simulink library "bcm"  (R2021b)
settings: Solver=VariableStepAuto  StartTime=0.0  StopTime=10.0  RelTol=1e-3
undefined symbols (not defined in the file or in its folder): ENUM_ANTITHEFT_ALARM, ENUM_ANTITHEFT_ARM, ENUM_ANTITHEFT_DISARM, ENUM_ANTITHEFT_WAIT, ENUM_GEARPOSNTOCAN_P, ENUM_PDKEYRAWLULOCK_INUNLOCK, ENUM_PDKEYRAWPS_INPS, ENUM_POWERSTA_READY, ENUM_POWERSTA_STANDBY, FALSE, KBCM_ALMBrightnessDark_enum, KBCM_AmbBlue_enum, KBCM_AmbBreathT_K, KBCM_AmbBreathTOut_K, KBCM_AmbGreen_enum, KBCM_AmbLightUser_enum, KBCM_AmbPreset_enum, KBCM_AmbRed_enum, KBCM_Antitheft_enum_ovrdflg, KBCM_Antitheft_enum_ovrdval, KBCM_APMDoorCtrlSta_flg_ovrdflg, KBCM_APMDoorCtrlSta_flg_ovrdval, KBCM_DelayTSW_flg, KBCM_DiagFLTC_mA, KBCM_DiagFMHT_s, KBCM_DiagFRTC_mA, KBCM_DiagRLTC_mA, KBCM_DiagRRTC_mA, KBCM_DrAPMRetryTimes_cnt, KBCM_DrOpenWdwOT_s, KBCM_DrOpenWdwReady_s, KBCM_ESSOffT_ms, KBCM_ESSOnT_ms, KBCM_IVIRstHoldT_ms, KBCM_IVIRstTriggerT_ms, KBCM_ONDelayT_ms, KBCM_ReDetectT_K, KBCM_RmLampKeep_min, KBCM_RmLpKeyInT_s, KBCM_RmLpKeyMissT_s, KBCM_SlpDebounceTime_s, KBCM_SPTGDetectT_sec, KBCM_SPTGLeave_flg, KBCM_SPTGLeftBound_cm, KBCM_SPTGLeftBoundOut_cm, KBCM_SPTGLowerBound_cm, KBCM_SPTGLowerBoundOut_cm, KBCM_SPTGRightBound_cm, KBCM_SPTGRightBoundOut_cm, KBCM_SPTGTOut_K, KBCM_SPTGUpperBound_cm, KBCM_SPTGUpperBoundOut_cm, KBCM_SPTGWaitDKC_sec, KBCM_USSDis_cm, KBCM_USSFilterT_K, KBCM_WaitAPMPwr_K, KBCM_WdwManualDetT_s, MIN2SEC, TRUE, XX2KXX
libraries: simulink x41, $bdroot x3, hcu_lib x2
(part 4 of 6)

== system bcm/BCM/BCM/FlasherSignal/Subsystem ==
  VINP_APSActive_flg : Inport
  VINP_AVMparkingmode_enum : Inport  Port=2
  Compare To Constant1 : simulink/Logic and Bit Operations/Compare To Constant  relop===  const=1  OutDataTypeStr=boolean
  Compare To Constant10 : simulink/Logic and Bit Operations/Compare To Constant  relop=>=  const=2  OutDataTypeStr=boolean
  Compare To Constant11 : simulink/Logic and Bit Operations/Compare To Constant  relop===  const=1  OutDataTypeStr=boolean
  Compare To Constant2 : simulink/Logic and Bit Operations/Compare To Constant  relop===  const=3  OutDataTypeStr=boolean
  Compare To Constant3 : simulink/Logic and Bit Operations/Compare To Constant  relop===  const=5  OutDataTypeStr=boolean
  Compare To Constant4 : simulink/Logic and Bit Operations/Compare To Constant  relop===  const=2  OutDataTypeStr=boolean
  Compare To Constant5 : simulink/Logic and Bit Operations/Compare To Constant  relop===  const=4  OutDataTypeStr=boolean
  Compare To Constant6 : simulink/Logic and Bit Operations/Compare To Constant  relop===  const=6  OutDataTypeStr=boolean
  Constant : Constant  OutDataTypeStr=uint8
  Constant1 : Constant  Value=0  OutDataTypeStr=uint8
  Constant2 : Constant  Value=2  OutDataTypeStr=uint8
  Constant3 : Constant  Value=0  OutDataTypeStr=uint8
  Constant7 : Constant  Value=0  OutDataTypeStr=uint8
  Detect Decrease : simulink/Logic and Bit Operations/Detect Decrease  vinit=0.0  OutDataTypeStr=boolean
  Detect Increase : simulink/Logic and Bit Operations/Detect Increase  vinit=0.0  OutDataTypeStr=boolean
  OR : Logic  Operator=OR  Inputs=3  AllPortsSameDT=off  OutDataTypeStr=boolean
  OR1 : Logic  Operator=OR  Inputs=3  AllPortsSameDT=off  OutDataTypeStr=boolean
  Sum : Sum  Inputs=|++
  Switch{,1..2,5} (4 alike) : Switch  Criteria=u2 > Threshold
  Unit Delay1 : UnitDelay  SampleTime=-1  HasFrameUpgradeWarning=on
  APS_LTurnReq : Outport
  APS_RTurnReq : Outport  Port=2
  wires:
  Compare To Constant2/1 -> OR/2
  Compare To Constant1/1 -> OR/1
  Compare To Constant3/1 -> OR/3
  Compare To Constant4/1 -> OR1/1
  Compare To Constant5/1 -> OR1/2
  Compare To Constant6/1 -> OR1/3
  Detect Increase/1 -> Switch/2
  OR/1 -> Switch1/2
  OR1/1 -> Switch2/2
  Constant/1 -> Switch1/1
  Constant1/1 -> Switch1/3
  Constant2/1 -> Switch2/1
  Constant3/1 -> Switch2/3
  Switch1/1 -> Sum/1
  Switch2/1 -> Sum/2
  Detect Decrease/1 -> Switch5/2
  Constant7/1 -> Switch5/1
  Switch5/1 -> Switch/3
  Unit Delay1/1 -> Switch5/3
  Switch/1 -> Compare To Constant10/1, Compare To Constant11/1, Unit Delay1/1
  Sum/1 -> Switch/1
  Compare To Constant10/1 -> APS_LTurnReq/1
  Compare To Constant11/1 -> APS_RTurnReq/1
  VINP_AVMparkingmode_enum/1 -> Compare To Constant6/1, Compare To Constant5/1, Compare To Constant4/1, Compare To Constant3/1, Compare To Constant2/1, Compare To Constant1/1
  VINP_APSActive_flg/1 -> Detect Decrease/1, Detect Increase/1

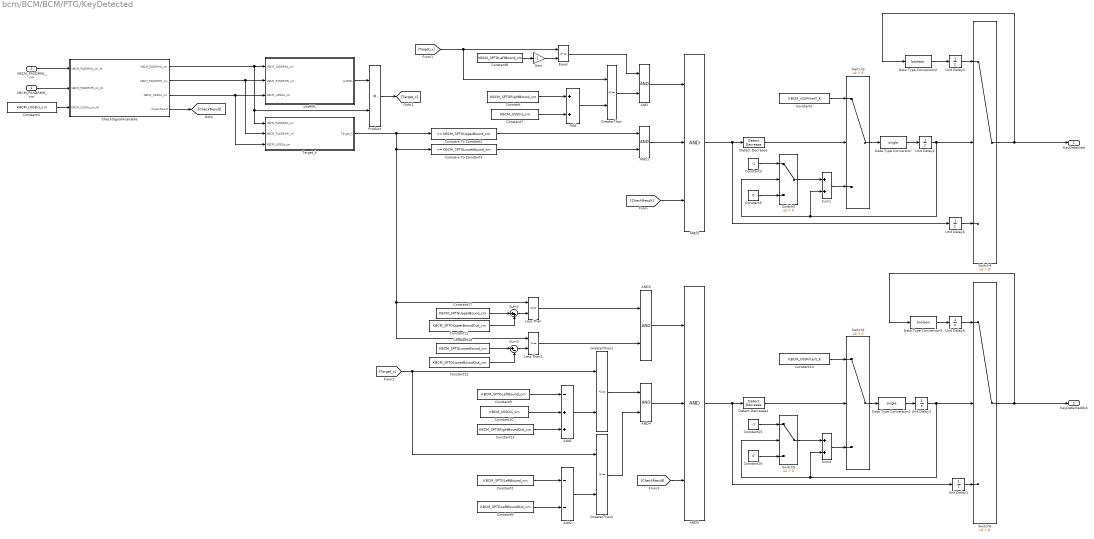
== system bcm/BCM/BCM/PTG/KeyDetected ==
  VBCM_PASDRMR_cm : Inport
  VBCM_PASDRML_cm : Inport  Port=2
  AND{,1,3..4} (4 alike) : Logic  AllPortsSameDT=off  OutDataTypeStr=boolean
  AND2 : Logic  Inputs=3  AllPortsSameDT=off  OutDataTypeStr=boolean
  AND5 : Logic  Inputs=3  AllPortsSameDT=off  OutDataTypeStr=boolean
  Add : Sum
  Add1 : Sum  Inputs=-++
  Add2 : Sum  Inputs=--
  CheckSignalAvailable : Subsystem
  Compare To Constant2 : simulink/Logic and Bit Operations/Compare To Constant  relop=<=  const=KBCM_SPTGUpperBound_cm  OutDataTypeStr=boolean
  Compare To Constant3 : simulink/Logic and Bit Operations/Compare To Constant  relop=>=  const=KBCM_SPTGLowerBound_cm  OutDataTypeStr=boolean
  Constant : Constant  Value=KBCM_SPTGRightBound_cm
  Constant1 : Constant  Value=KBCM_USSFilterT_K
  Constant10 : Constant  Value=KBCM_USSDis_cm
  Constant11 : Constant  Value=KBCM_SPTGUpperBoundOut_cm
  Constant12 : Constant  Value=KBCM_SPTGLowerBoundOut_cm
  Constant13 : Constant  Value=KBCM_SPTGRightBoundOut_cm
  Constant14 : Constant  Value=KBCM_USSFilterT_K
  Constant15 : Constant  Value=-1  OutDataTypeStr=single
  Constant16 : Constant  Value=0  OutDataTypeStr=single
  Constant17 : Constant  Value=KBCM_SPTGUpperBound_cm
  Constant18 : Constant  Value=KBCM_SPTGLowerBound_cm
  Constant2 : Constant  Value=KBCM_SPTGLeftBound_cm
  Constant3 : Constant  Value=-1  OutDataTypeStr=single
  Constant4 : Constant  Value=KBCM_USSDis_cm
  Constant5 : Constant  Value=0  OutDataTypeStr=single
  Constant6 : Constant  Value=KBCM_SPTGLeftBoundOut_cm
  Constant7 : Constant  Value=KBCM_USSDis_cm
  Constant8 : Constant  Value=KBCM_SPTGLeftBound_cm
  Constant9 : Constant  Value=KBCM_SPTGLeftBound_cm
  Data Type Conversion : DataTypeConversion  OutDataTypeStr=single
  Data Type Conversion1 : DataTypeConversion  OutDataTypeStr=single
  Data Type Conversion2 : DataTypeConversion  OutDataTypeStr=boolean
  Data Type Conversion3 : DataTypeConversion  OutDataTypeStr=boolean
  Detect Decrease : simulink/Logic and Bit Operations/Detect Decrease  vinit=0.0  OutDataTypeStr=boolean
  Detect Decrease1 : simulink/Logic and Bit Operations/Detect Decrease  vinit=0.0  OutDataTypeStr=boolean
  Equal : RelationalOperator  OutDataTypeStr=boolean  RndMeth=Simplest
  Gain : Gain  Gain=-1
  GreaterThan : RelationalOperator  Operator=<=  OutDataTypeStr=boolean  RndMeth=Simplest
  GreaterThan1 : RelationalOperator  Operator=<=  OutDataTypeStr=boolean  RndMeth=Simplest
  GreaterThan2 : RelationalOperator  OutDataTypeStr=boolean  RndMeth=Simplest
  Less Than : RelationalOperator  Operator=<=  OutDataTypeStr=boolean  RndMeth=Simplest
  Less Than1 : RelationalOperator  OutDataTypeStr=boolean  RndMeth=Simplest
  Product : Product
  Sum1 : Sum
  Sum2 : Sum  Inputs=|++
  Sum3 : Sum  Inputs=|+-
  Sum4 : Sum
  Switch{1..6} (6 alike) : Switch  Criteria=u2 > Threshold
  Target_h : Subsystem
  Unit Delay{1..6} (6 alike) : UnitDelay  SampleTime=-1  HasFrameUpgradeWarning=on
  cosRML : Subsystem
  KeyDetected : Outport
  KeyDetectedOut : Outport  Port=2
  wires:
  Constant4/1 -> CheckSignalAvailable/3(KBCM_USSDis_cm_IN)
  CheckSignalAvailable/1(VBCM_PASDRML_cm) -> cosRML/1(VBCM_PASDRML_cm), Target_h/1(VBCM_PASDRML_cm), Product/2
  CheckSignalAvailable/2(VBCM_PASDRMR_cm) -> Target_h/2(VBCM_PASDRMR_cm), cosRML/2(VBCM_PASDRMR_cm)
  CheckSignalAvailable/3(KBCM_USSDis_cm) -> Target_h/3(KBCM_USSDis_cm), cosRML/3(KBCM_USSDis_cm)
  Target_h/1(Target_h) -> Less Than1/1, Less Than/1, Compare To Constant3/1, Compare To Constant2/1
  Compare To Constant2/1 -> AND1/1
  Compare To Constant3/1 -> AND1/2
  AND1/1 -> AND2/2
  AND/1 -> AND2/1
  cosRML/1(cosRML) -> Product/1
  CheckSignalAvailable/4(CheckResult) -> [CheckResult]
  [CheckResult] -> AND2/3
  Detect Decrease/1 -> Switch2/2
  Switch2/1 -> Data Type Conversion/1
  Constant1/1 -> Switch2/1
  Sum1/1 -> Switch2/3
  Unit Delay2/1 -> Switch3/2, Sum1/2, Switch4/2
  Constant3/1 -> Switch3/1
  Constant5/1 -> Switch3/3
  Switch3/1 -> Sum1/1
  Switch4/1 -> Data Type Conversion2/1, KeyDetected/1
  Unit Delay4/1 -> Switch4/1
  VBCM_PASDRML_cm/1 -> CheckSignalAvailable/1(VBCM_PASDRML_cm_IN)
  VBCM_PASDRMR_cm/1 -> CheckSignalAvailable/2(VBCM_PASDRMR_cm_IN)
  AND2/1 -> Unit Delay6/1, Detect Decrease/1
  GreaterThan1/1 -> AND4/1
  Add1/1 -> GreaterThan1/2
  [Target_x] -> GreaterThan2/1, GreaterThan1/1
  Product/1 -> [Target_x]
  [Target_x] -> GreaterThan/1, Equal/1
  Constant17/1 -> Sum2/1
  Constant11/1 -> Sum2/2
  Constant12/1 -> Sum3/2
  Constant18/1 -> Sum3/1
  [CheckResult] -> AND5/3
  AND3/1 -> AND5/1
  AND4/1 -> AND5/2
  AND5/1 -> Unit Delay1/1, Detect Decrease1/1
  Unit Delay5/1 -> Switch6/1
  Switch6/1 -> KeyDetectedOut/1, Data Type Conversion3/1
  Switch5/1 -> Sum4/1
  Constant16/1 -> Switch5/3
  Constant15/1 -> Switch5/1
  Unit Delay3/1 -> Switch6/2, Sum4/2, Switch5/2
  Sum4/1 -> Switch1/3
  Constant14/1 -> Switch1/1
  Switch1/1 -> Data Type Conversion1/1
  Detect Decrease1/1 -> Switch1/2
  Sum2/1 -> Less Than/2
  Less Than/1 -> AND3/1
  Sum3/1 -> Less Than1/2
  Less Than1/1 -> AND3/2
  Constant10/1 -> Add1/2
  Constant9/1 -> Add1/1
  Constant13/1 -> Add1/3
  Constant7/1 -> Add/2
  Equal/1 -> AND/1
  GreaterThan/1 -> AND/2
  Constant/1 -> Add/1
  Add/1 -> GreaterThan/2
  GreaterThan2/1 -> AND4/2
  Constant2/1 -> Add2/1
  Constant6/1 -> Add2/2
  Add2/1 -> GreaterThan2/2
  Unit Delay1/1 -> Switch6/3
  Unit Delay6/1 -> Switch4/3
  Constant8/1 -> Gain/1
  Gain/1 -> Equal/2
  Data Type Conversion/1 -> Unit Delay2/1
  Data Type Conversion1/1 -> Unit Delay3/1
  Data Type Conversion2/1 -> Unit Delay4/1
  Data Type Conversion3/1 -> Unit Delay5/1

== system bcm/BCM/BCM/PTG/Subsystem1 ==
  VAPM_PASDRMR_cm : Inport
  Add4 : Sum
  Compare To Constant1 : simulink/Logic and Bit Operations/Compare To Constant  relop=~=  const=0  OutDataTypeStr=boolean
  Compare To Constant6 : simulink/Logic and Bit Operations/Compare To Constant  relop===  const=0  OutDataTypeStr=boolean
  Compare To Constant8 : simulink/Logic and Bit Operations/Compare To Constant  relop===  const=255  OutDataTypeStr=boolean
  Constant1 : Constant  Value=0  OutDataTypeStr=uint8
  Constant12 : Constant  OutDataTypeStr=uint8
  Constant13 : Constant  Value=0  OutDataTypeStr=uint8
  Constant2 : Constant  OutDataTypeStr=uint8
  Constant3 : Constant  Value=KBCM_SPTGTOut_K
  Constant4 : Constant  Value=255  OutDataTypeStr=uint8
  Constant5 : Constant  Value=KBCM_SPTGTOut_K
  Detect Change : simulink/Logic and Bit Operations/Detect Change  vinit=0  OutDataTypeStr=boolean
  Equal : RelationalOperator  OutDataTypeStr=boolean  RndMeth=Simplest
  Equal1 : RelationalOperator  Operator===  OutDataTypeStr=boolean  RndMeth=Simplest
  Equal2 : RelationalOperator  Operator=~=  OutDataTypeStr=boolean  RndMeth=Simplest
  Logical Operator : Logic  Inputs=3  AllPortsSameDT=off  OutDataTypeStr=boolean
  Logical Operator2 : Logic  Operator=OR  AllPortsSameDT=off  OutDataTypeStr=boolean
  Switch{2..3,8..9} (4 alike) : Switch  Criteria=u2 > Threshold
  Unit Delay2 : UnitDelay  SampleTime=-1  HasFrameUpgradeWarning=on
  Unit Delay6 : UnitDelay  SampleTime=-1  HasFrameUpgradeWarning=on
  PASDRMR : Outport
  wires:
  Equal1/1 -> Logical Operator2/2
  Switch9/1 -> Add4/1
  Constant5/1 -> Equal1/1, Equal2/2
  Unit Delay6/1 -> Equal/1, Add4/2
  Compare To Constant8/1 -> Switch8/2
  Equal2/1 -> Logical Operator2/1
  Constant4/1 -> Switch3/3
  Switch2/1 -> Switch3/1, Unit Delay2/1
  Compare To Constant1/1 -> Logical Operator/2
  Logical Operator/1 -> Switch2/2
  Constant13/1 -> Switch9/1
  Add4/1 -> Switch8/1
  Unit Delay2/1 -> Switch2/3
  Constant12/1 -> Switch9/3
  Equal/1 -> Switch9/2
  Constant3/1 -> Equal/2
  Detect Change/1 -> Logical Operator/1
  Compare To Constant6/1 -> Logical Operator/3
  Constant1/1 -> Switch8/3
  Switch3/1 -> PASDRMR/1
  VAPM_PASDRMR_cm/1 -> Switch2/1, Detect Change/1, Compare To Constant1/1, Compare To Constant8/1
  Logical Operator2/1 -> Switch3/2
  Constant2/1 -> Equal1/2
  Switch8/1 -> Unit Delay6/1, Compare To Constant6/1, Equal2/1

== system bcm/BCM/BCM/PTG/Subsystem3 ==
  VAPM_PASDRML_cm : Inport
  Add4 : Sum
  Compare To Constant1 : simulink/Logic and Bit Operations/Compare To Constant  relop=~=  const=0  OutDataTypeStr=boolean
  Compare To Constant6 : simulink/Logic and Bit Operations/Compare To Constant  relop===  const=0  OutDataTypeStr=boolean
  Compare To Constant8 : simulink/Logic and Bit Operations/Compare To Constant  relop===  const=255  OutDataTypeStr=boolean
  Constant1 : Constant  Value=0  OutDataTypeStr=uint8
  Constant12 : Constant  OutDataTypeStr=uint8
  Constant13 : Constant  Value=0  OutDataTypeStr=uint8
  Constant2 : Constant  Value=0  OutDataTypeStr=uint8
  Constant3 : Constant  Value=KBCM_SPTGTOut_K
  Constant4 : Constant  Value=255  OutDataTypeStr=uint8
  Constant5 : Constant  Value=KBCM_SPTGTOut_K
  Detect Change : simulink/Logic and Bit Operations/Detect Change  vinit=0  OutDataTypeStr=boolean
  Equal : RelationalOperator  OutDataTypeStr=boolean  RndMeth=Simplest
  Equal1 : RelationalOperator  Operator===  OutDataTypeStr=boolean  RndMeth=Simplest
  Equal2 : RelationalOperator  Operator=~=  OutDataTypeStr=boolean  RndMeth=Simplest
  Logical Operator : Logic  Inputs=3  AllPortsSameDT=off  OutDataTypeStr=boolean
  Logical Operator2 : Logic  Operator=OR  AllPortsSameDT=off  OutDataTypeStr=boolean
  Switch{2..3,8..9} (4 alike) : Switch  Criteria=u2 > Threshold
  Unit Delay2 : UnitDelay  SampleTime=-1  HasFrameUpgradeWarning=on
  Unit Delay6 : UnitDelay  SampleTime=-1  HasFrameUpgradeWarning=on
  PASDRML : Outport
  wires:
  Constant2/1 -> Equal1/2
  Logical Operator2/1 -> Switch3/2
  VAPM_PASDRML_cm/1 -> Compare To Constant8/1, Compare To Constant1/1, Detect Change/1, Switch2/1
  Switch3/1 -> PASDRML/1
  Constant1/1 -> Switch8/3
  Compare To Constant6/1 -> Logical Operator/3
  Detect Change/1 -> Logical Operator/1
  Constant3/1 -> Equal/2
  Equal/1 -> Switch9/2
  Constant12/1 -> Switch9/3
  Unit Delay2/1 -> Switch2/3
  Add4/1 -> Switch8/1
  Constant13/1 -> Switch9/1
  Switch8/1 -> Equal2/1, Compare To Constant6/1, Unit Delay6/1
  Logical Operator/1 -> Switch2/2
  Compare To Constant1/1 -> Logical Operator/2
  Switch2/1 -> Unit Delay2/1, Switch3/1
  Constant4/1 -> Switch3/3
  Equal2/1 -> Logical Operator2/1
  Compare To Constant8/1 -> Switch8/2
  Unit Delay6/1 -> Add4/2, Equal/1
  Constant5/1 -> Equal2/2, Equal1/1
  Switch9/1 -> Add4/1
  Equal1/1 -> Logical Operator2/2

== system bcm/BCM/BCM/PTG/KeyDetected/CheckSignalAvailable ==
  VBCM_PASDRML_cm_IN : Inport
  VBCM_PASDRMR_cm_IN : Inport  Port=2
  KBCM_USSDis_cm_IN : Inport  Port=3
  AND : Logic  Inputs=3  AllPortsSameDT=off  OutDataTypeStr=boolean
  Constant : Constant  OutDataTypeStr=single
  Constant1 : Constant  OutDataTypeStr=single
  Constant2 : Constant  OutDataTypeStr=single
  Constant3 : Constant  Value=KBCM_SPTGLowerBound_cm
  Constant4 : Constant  Value=KBCM_SPTGLowerBoundOut_cm
  Constant5 : Constant  Value=KBCM_SPTGLowerBound_cm
  Constant6 : Constant  Value=KBCM_SPTGLowerBoundOut_cm
  Demux : Demux  Outputs=3
  Equal : RelationalOperator  OutDataTypeStr=boolean  RndMeth=Simplest
  Equal1 : RelationalOperator  OutDataTypeStr=boolean  RndMeth=Simplest
  GreaterThan : RelationalOperator  OutDataTypeStr=boolean  RndMeth=Simplest
  Max : MinMax  Function=max  Inputs=3
  Mux : Mux  Inputs=3
  Mux1 : Mux  Inputs=3
  Sum : Sum  Inputs=+-
  Sum1 : Sum  Inputs=+++
  Sum2 : Sum  Inputs=|+-
  Sum3 : Sum  Inputs=|+-
  Switch : Switch  Criteria=u2 > Threshold
  VBCM_PASDRML_cm : Outport
  VBCM_PASDRMR_cm : Outport  Port=2
  KBCM_USSDis_cm : Outport  Port=3
  CheckResult : Outport  Port=4
  wires:
  GreaterThan/1 -> AND/1
  VBCM_PASDRML_cm_IN/1 -> [VBCM_PASDRML_cm_IN]
  VBCM_PASDRMR_cm_IN/1 -> [VBCM_PASDRMR_cm_IN]
  KBCM_USSDis_cm_IN/1 -> [KBCM_USSDis_cm_IN]
  AND/1 -> Switch/2, CheckResult/1
  Mux/1 -> Switch/1
  [VBCM_PASDRML_cm_IN] -> Mux/1
  [VBCM_PASDRMR_cm_IN] -> Mux/2
  [KBCM_USSDis_cm_IN] -> Mux/3
  Mux1/1 -> Switch/3
  Constant/1 -> Mux1/1
  Constant1/1 -> Mux1/2
  Switch/1 -> Demux/1
  Demux/1 -> VBCM_PASDRML_cm/1
  Demux/2 -> VBCM_PASDRMR_cm/1
  Demux/3 -> KBCM_USSDis_cm/1
  Equal/1 -> AND/2
  [VBCM_PASDRML_cm_IN] -> Max/1, Sum1/1
  [VBCM_PASDRMR_cm_IN] -> Max/2, Sum1/2
  [KBCM_USSDis_cm_IN] -> Max/3, Sum1/3
  Sum1/1 -> Sum/1
  Max/1 -> Sum/2, GreaterThan/2
  Sum/1 -> GreaterThan/1
  Constant2/1 -> Mux1/3
  Equal1/1 -> AND/3
  [VBCM_PASDRMR_cm_IN] -> Equal/1
  Constant3/1 -> Sum2/1
  Constant4/1 -> Sum2/2
  Sum2/1 -> Equal/2
  Sum3/1 -> Equal1/2
  Constant6/1 -> Sum3/2
  Constant5/1 -> Sum3/1
  [VBCM_PASDRML_cm_IN] -> Equal1/1

== system bcm/BCM/BCM/PTG/KeyDetected/Target_h ==
  VBCM_PASDRML_cm : Inport
  VBCM_PASDRMR_cm : Inport  Port=2
  KBCM_USSDis_cm : Inport  Port=3
  Data Type Conversion : DataTypeConversion
  Divide : Product  Inputs=*/
  Gain : Gain  Gain=2
  Gain1 : Gain  Gain=0.5
  Product : Product  Inputs=4
  Sqrt1 : Sqrt  SaturateOnIntegerOverflow=on
  Sum : Sum  Inputs=+-
  Sum1 : Sum  Inputs=+++
  Sum2 : Sum  Inputs=+-
  Sum3 : Sum  Inputs=+-
  Terminator : Terminator
  Target_h : Outport
  wires:
  Divide/1 -> Data Type Conversion/1, Target_h/1
  VBCM_PASDRML_cm/1 -> Sum/2, Sum1/1
  VBCM_PASDRMR_cm/1 -> Sum2/2, Sum1/2
  KBCM_USSDis_cm/1 -> Divide/2, Sum3/2, Sum1/3
  Sum1/1 -> Gain1/1
  Sum/1 -> Product/2
  Sum2/1 -> Product/3
  Sum3/1 -> Product/4
  Product/1 -> Sqrt1/1
  Sqrt1/1 -> Gain/1
  Gain/1 -> Divide/1
  Gain1/1 -> Sum3/1, Sum2/1, Sum/1, Product/1
  Data Type Conversion/1 -> Terminator/1  "VBCM_Targeth_cm"

== system bcm/BCM/BCM/PTG/KeyDetected/cosRML ==
  VBCM_PASDRML_cm : Inport
  VBCM_PASDRMR_cm : Inport  Port=2
  KBCM_USSDis_cm : Inport  Port=3
  Divide : Product  Inputs=*/
  Gain : Gain  Gain=2
  Product : Product
  Square : Math  Operator=square  SaturateOnIntegerOverflow=on
  Square1 : Math  Operator=square  SaturateOnIntegerOverflow=on
  Square2 : Math  Operator=square  SaturateOnIntegerOverflow=on
  Sum : Sum  Inputs=+-+
  cosRML : Outport
  wires:
  VBCM_PASDRML_cm/1 -> Product/1, Square/1
  VBCM_PASDRMR_cm/1 -> Square1/1
  KBCM_USSDis_cm/1 -> Product/2, Square2/1
  Square/1 -> Sum/1
  Square1/1 -> Sum/2
  Square2/1 -> Sum/3
  Product/1 -> Gain/1
  Sum/1 -> Divide/1
  Divide/1 -> cosRML/1
  Gain/1 -> Divide/2

== stateflow chart bcm/BCM/BCM/AntiTheft/Chart ==
  settings: sampleTime=StepSize
  state ATCtrl [parallel]
    settings: executionOrder=5
    state StandBy
      en:VBCM_ATCtrl_enum=0;
    state Lock
      en:VBCM_ATCtrl_enum=1;
    note: 350 ms
    state Unlock
      en:VBCM_ATCtrl_enum=2;
    (default) -> ATCtrl.StandBy
    ATCtrl.StandBy -> ATCtrl.Lock [order 1] : eLampLock
    ATCtrl.Lock -> ATCtrl.StandBy [order 1] : [after(35,tick)]
    ATCtrl.Unlock -> ATCtrl.Lock [order 2] : eLampLock
    ATCtrl.Lock -> ATCtrl.Unlock [order 2] : eLampUnlock
    ATCtrl.StandBy -> ATCtrl.Unlock [order 2] : eLampUnlock
    ATCtrl.Unlock -> ATCtrl.StandBy [order 1] : [after(35,tick)]
  state AlertTone [parallel]
    settings: executionOrder=11
    state OFF
      en:VBCM_LockAlarm_enum=0;
    state Lock_Success
      en:VBCM_LockAlarm_enum=1;
    (default) -> OFF
    Lock_Success -> OFF : [after(5,tick)]
    AlertTone -> Lock_Success : eLockAlert [IVI_Lock_SoundSW_Sta==1]
  state Main [parallel]
    settings: executionOrder=1
    state sDisarm
      en:AntitheftSta=0;
      fFirst=1;
    state sSecurity
      state sSecurity
        en:
        AntitheftSta=1;
        fFirst=0;
      note: 28 sec
      note: 10 times
      state sAlarm
        en:
        AntitheftSta=3;
        ATAlarm=1;
        Horn.eHornAlarm;
        CountAlarm=CountAlarm+1;
        ex:ATAlarm=0;
      (junction 1705) -> (junction 1971) [order 2] : {Horn.eHornLock;}
      (junction 1705) -> Main.sSecurity.sSecurity [order 1] : [fHornOFF==1||fFirst==1]
          | /{fHornOFF=0;AlertTone.eLockAlert;}
      (junction 1971) -> Main.sSecurity.sSecurity
      Main.sSecurity.sSecurity -> sAlarm : eDoorOpen[CountAlarm<10]
      sAlarm -> Main.sSecurity.sSecurity : [after(2800,tick)]
    note: 1 sec
    state sLockCheck
    (default) -> (junction 2132) : {CountAlarm = VINP_FlashCountAlarm_enum;}
    (junction 2132) -> (junction 2133) [order 1]
    (junction 2133) -> (junction 2135) [order 1]
    (junction 2132) -> sDisarm [order 2]
    (junction 2133) -> Main.sSecurity.sSecurity [order 2] : [VBCM_FlashAntitheft_enum == ENUM_ANTITHEFT_ARM]
    (junction 2135) -> sAlarm : [VBCM_FlashAntitheft_enum == ENUM_ANTITHEFT_ALARM]
    (junction 1713) -> sDisarm : {ATLockCtrl.eActUnlock;Horn.eLockFail;}
    (junction 1703) -> (junction 1713) [order 1] : [!DrLockSta||AllDoorSW||TailgateSW||HoodSW]
    (junction 1703) -> (junction 1705) [order 2] : {CountAlarm=0;}
    (junction 1686) -> (junction 1713) [order 1] : [AllDoorSW||TailgateSW||HoodSW]
    sLockCheck -> (junction 1703) : [after(100,tick)]
    sDisarm -> sDisarm [order 2] : eUnlock{ATCtrl.eLampUnlock;ATLockCtrl.eActUnlock;}
    (junction 1686) -> sLockCheck [order 2] : {ATLockCtrl.eActLock;}
    (junction 1712) -> (junction 1686) : {ATCtrl.eLampLock;}
    sDisarm -> (junction 1712) [order 1] : eLock
    Main.sSecurity -> (junction 1712) [order 2] : eLock
    Main.sSecurity -> sDisarm [order 1] : eUnlock{ATCtrl.eLampUnlock;ATLockCtrl.eActUnlock;}
    Main.sSecurity -> sDisarm [order 3] : eForceDisarm
  state DKCCmd [parallel]
    settings: executionOrder=2
    state WaitForZone
    state Lock
      en:Main.eLock;
    state Unlock
      en:Main.eUnlock;
    state sStandBy
    state Tailgate
      en:DoorSWDetection.TailgateSW.eTailgate;
      PowerTailgate.eTailgateRemote;
    state FindCar
      en:Horn.eHornLock;ATCtrl.eLampUnlock;
    state TailgateLockFail
      en:Horn.eLockFail;Main.eUnlock;
    state TailgateHandle
      en:DoorSWDetection.TailgateSW.eTailgate;
      PowerTailgate.eTailgateHandle;
    state ForceDisarm
      en:Main.eForceDisarm;
    state FindCarMute
      en:ATCtrl.eLampUnlock;
    DKCCmd -> (junction 2148) : [hasChanged(P_CommandtoBCM)]{PcmdBuf=P_CommandtoBCM;}
    (junction 2148) -> DKCCmd.WaitForZone [order 2]
    (junction 2148) -> (junction 2154) [order 1]
    DKCCmd.WaitForZone -> (junction 2154) [order 2]
    (junction 2154) -> (junction 2045) : [VINP_CANMsgValidGWZoneDR1_flg&&VINP_CANMsgValidGWZoneFR1_flg]
    DKCCmd.WaitForZone -> (junction 2151) [order 1] : [after(150,tick)]
    (junction 2151) -> (junction 2045)
    (junction 2045) -> DKCCmd.Lock [order 1] : [VehSpeed<=0&&PcmdBuf==1]
    (junction 2045) -> (junction 2046) [order 2]
    (default) -> DKCCmd.sStandBy : {PcmdBuf=0;}
    (junction 2046) -> DKCCmd.Unlock [order 1] : [VehSpeed<=0&&PcmdBuf==2]
    (junction 2046) -> (junction 2047) [order 2]
    (junction 2047) -> DKCCmd.Tailgate [order 1] : [PcmdBuf==3]
    (junction 2047) -> (junction 2048) [order 2]
    (junction 2048) -> DKCCmd.FindCar [order 1] : [PcmdBuf==4]
    (junction 2048) -> (junction 2049) [order 2]
    (junction 2049) -> TailgateLockFail [order 1] : [PcmdBuf==5]
    (junction 2049) -> (junction 2050) [order 2]
    (junction 2050) -> DKCCmd.TailgateHandle [order 1] : [PcmdBuf==6]
    (junction 2050) -> (junction 2108) [order 2]
    (junction 2108) -> ForceDisarm [order 1] : [PcmdBuf==7]
    (junction 2108) -> (junction 2124) [order 2]
    (junction 2124) -> DKCCmd.sStandBy [order 2]
    (junction 2124) -> DKCCmd.FindCarMute [order 1] : [PcmdBuf==8]
  state DoorSWDetection [parallel]
    settings: executionOrder=4
    state DrDoor [parallel]
      settings: executionOrder=1
      state DrDoorSW_Open
      state DrDoorSW_Close
      (default) -> DrDoorSW_Open
      DrDoorSW_Open -> DrDoorSW_Close : [!DrDoorSW]
      DrDoorSW_Close -> DrDoorSW_Open : [DrDoorSW]/{Main.eDoorOpen;}
    state PsDoor [parallel]
      settings: executionOrder=2
      state PsDoorSW_Open
      state PsDoorSW_Close
      (default) -> PsDoorSW_Open
      PsDoorSW_Open -> PsDoorSW_Close : [!PsDoorSW]
      PsDoorSW_Close -> PsDoorSW_Open : [PsDoorSW]/{Main.eDoorOpen;}
    state RLDoor [parallel]
      settings: executionOrder=3
      state RLDoorSW_Open
      state RLDoorSW_Close
      (default) -> RLDoorSW_Open
      RLDoorSW_Open -> RLDoorSW_Close : [!RLDoorSW]
      RLDoorSW_Close -> RLDoorSW_Open : [RLDoorSW]/{Main.eDoorOpen;}
    state RRDoor [parallel]
      settings: executionOrder=4
      state RRDoorSW_Open
      state RRDoorSW_Close
      (default) -> RRDoorSW_Open
      RRDoorSW_Open -> RRDoorSW_Close : [!RRDoorSW]
      RRDoorSW_Close -> RRDoorSW_Open : [RRDoorSW]/{Main.eDoorOpen;}
    state HoodSW [parallel]
      settings: executionOrder=5
      state HoodSW_Open
      state HoodSW_Close
      (default) -> HoodSW_Open
      HoodSW_Open -> HoodSW_Close : [!HoodSW]
      HoodSW_Close -> HoodSW_Open : [HoodSW]/{Main.eDoorOpen;}
    state TailgateSW [parallel]
      settings: executionOrder=6
      state TailgateSW_Open
      state TailgateSW_Close
      state sRemote
      state Ignore
      (default) -> TailgateSW_Open
      TailgateSW_Open -> TailgateSW_Close : [!TailgateSW]
      TailgateSW_Close -> TailgateSW_Open [order 1] : [TailgateSW]/{Main.eDoorOpen;}
      TailgateSW_Close -> sRemote [order 2] : eTailgate
      (junction 1886) -> TailgateSW_Close [order 2] : [after(1500,tick)]
      Ignore -> TailgateSW_Close : [!TailgateSW]
      sRemote -> (junction 1886)
      (junction 1886) -> Ignore [order 1] : [TailgateSW]
    note: 15 sec
  state Horn [parallel]
    settings: executionOrder=3
    state sStandBy
      en:HornCtrl=0;
    note: 250 ms
    state sAlarm2
      en:HornCtrl=0;
    state sAlarm1
      en:HornCtrl=1;
    state sLock
      en:HornCtrl=1;
    state sKeyIN1
      en:HornCtrl=1;
    state sKeyIN2
      en:HornCtrl=0;
    state sLockFail1
      en:HornCtrl=1;
    state sLockFail2
      en:HornCtrl=0;
    state sLockFail3
      en:HornCtrl=1;
    (default) -> Horn.sStandBy
    (junction 1821) -> Horn.sStandBy
    sAlarm1 -> sAlarm2 : [after(25,tick)]
    sAlarm2 -> (junction 1821) [order 1] : [ATAlarm==0]
    Horn -> sAlarm1 [order 1] : eHornAlarm
    (junction 1827) -> (junction 1821)
    sAlarm2 -> sAlarm1 [order 2] : [after(25,tick)]
    sLock -> (junction 1827) : [after(3,tick)]
    (junction 2026) -> (junction 1827)
    Horn -> sLock [order 2] : eHornLock
    sKeyIN2 -> sLock : [after(5,tick)]
    Horn -> sKeyIN1 [order 3] : eKeyIN
    sKeyIN1 -> sKeyIN2 : [after(3,tick)]
    Horn -> sLockFail1 [order 4] : eLockFail
    sLockFail1 -> sLockFail2 : [after(10,tick)]
    sLockFail2 -> sLockFail3 : [after(30,tick)]
    sLockFail3 -> (junction 2026) : [after(10,tick)]
  state ATLockCtrl [parallel]
    settings: executionOrder=6
    state Lock
      en:ATLockCtrl=1;
    state StandBy
      en:ATLockCtrl=0;
    note: 350 ms
    state Unlock
      en:ATLockCtrl=2;
    (default) -> ATLockCtrl.StandBy
    ATLockCtrl.StandBy -> ATLockCtrl.Lock [order 1] : eActLock
    ATLockCtrl.Lock -> ATLockCtrl.StandBy : [after(35,tick)]
    ATLockCtrl.Unlock -> ATLockCtrl.Lock [order 2] : eActLock
    ATLockCtrl.StandBy -> ATLockCtrl.Unlock [order 2] : eActUnlock
    ATLockCtrl.Unlock -> ATLockCtrl.StandBy [order 1] : [after(35,tick)]
  state VIGCommand [parallel]
    settings: executionOrder=7
    state WaitForZone
    state StandBy
    state Lock
      en:Main.eLock;
    state Unlock
      en:Main.eUnlock;
    state FindCar
      en:Horn.eHornLock;ATCtrl.eLampUnlock;
    state FindCarMute
      en:ATCtrl.eLampUnlock;
    state Tailgate
      en:DoorSWDetection.TailgateSW.eTailgate;
      PowerTailgate.eTailgateRemote;
    state TailgateReject
      en:PowerTailgate.eTailgateReject;
    (default) -> VIGCommand.WaitForZone
    VIGCommand.WaitForZone -> VIGCommand.StandBy : [VINP_CANMsgValidGWZoneDR1_flg&&VINP_CANMsgValidGWZoneFR1_flg]
    VIGCommand.StandBy -> VIGCommand.Lock [order 1] : [VehSpeed<=0&&(VIG_Cmd==1||VIG_Cmd==5)]
    VIGCommand.Lock -> VIGCommand.StandBy : [VIG_Cmd==0]
    (junction 1941) -> VIGCommand.Lock [order 1] : [AntitheftSta==0||AntitheftSta==2]/{fHornOFF=1;}
    VIGCommand.StandBy -> (junction 1941) [order 6] : [VehSpeed<=0&&VIG_Cmd==7]
    (junction 1941) -> VIGCommand.Unlock [order 2] : [fVIGHandle==0]
    VIGCommand.StandBy -> VIGCommand.Unlock [order 2] : [VehSpeed<=0&&(VIG_Cmd==2||VIG_Cmd==6)]
    VIGCommand.Unlock -> VIGCommand.StandBy : [VIG_Cmd==0]
    VIGCommand.StandBy -> VIGCommand.FindCar [order 3] : [VIG_Cmd==3]
    VIGCommand.FindCar -> VIGCommand.StandBy : [VIG_Cmd==0]
    VIGCommand.StandBy -> VIGCommand.FindCarMute [order 5] : [VIG_Cmd==8]
    VIGCommand.FindCarMute -> VIGCommand.StandBy : [VIG_Cmd==0]
    VIGCommand.Tailgate -> VIGCommand.StandBy : [VIG_Cmd==0]
    (junction 2118) -> VIGCommand.Tailgate
    (junction 2116) -> (junction 2118) [order 2]
    VIGCommand.StandBy -> (junction 2116) [order 4] : [VIG_Cmd==4]
    (junction 2116) -> TailgateReject [order 1] : [PwrSta==5]
    TailgateReject -> VIGCommand.StandBy : [VIG_Cmd==0]
  state PowerTailgate [parallel]
    settings: executionOrder=9
    state StandBy
      en:TailgateRemote=0;
    state TailgateRemote
      en:TailgateRemote=1;
    note: 200 ms
    state TailgateHandle
      en:TailgateRemote=2;
    note: 200 ms
    state TailgateHandle1
      en:TailgateRemote=3;
    (default) -> PowerTailgate.StandBy
    PowerTailgate.StandBy -> TailgateRemote [order 1] : eTailgateRemote
    TailgateRemote -> PowerTailgate.StandBy : [after(20,tick)]
    PowerTailgate.StandBy -> PowerTailgate.TailgateHandle [order 2] : eTailgateHandle
    PowerTailgate.TailgateHandle -> PowerTailgate.StandBy : [after(20,tick)]
    PowerTailgate.StandBy -> TailgateHandle1 [order 3] : eTailgateReject
    TailgateHandle1 -> PowerTailgate.StandBy : [after(20,tick)]
  state AGSTailgateOpen [parallel]
    settings: executionOrder=8
    state sStandBy
    state Tailgate
      en:DoorSWDetection.TailgateSW.eTailgate;
      PowerTailgate.eTailgateRemote;
    (default) -> AGSTailgateOpen.sStandBy
    AGSTailgateOpen.sStandBy -> AGSTailgateOpen.Tailgate : [APSOpenPTG==1&&TailgateSW==0]
    AGSTailgateOpen.Tailgate -> AGSTailgateOpen.sStandBy : [APSOpenPTG==0]
  state AntitheftSeat [parallel]
    settings: executionOrder=10
    state StandBy
      en:AntitheftSeatFlod=0;
    state Lock_Check
      en:AntitheftSeatFlod=0;
    state Flod
      en:AntitheftSeatFlod=1;
    note: 200 ms
    (default) -> AntitheftSeat.StandBy
    AntitheftSeat.StandBy -> Lock_Check : [fHornOFF==1]
    Lock_Check -> Flod : [fHornOFF==0]
    Flod -> Lock_Check [order 2] : [fHornOFF==1]
    Flod -> AntitheftSeat.StandBy [order 1] : [after(20,tick)]
  data: P_CommandtoBCM input uint8 [0..11]; PwrSta input uint8 [0..5]; ATLockCtrl output uint8; AllDoorSW input boolean [0..1]; HoodSW input boolean; TailgateSW input boolean; DrDoorSW input boolean; PsDoorSW input boolean; RLDoorSW input boolean; RRDoorSW input boolean; DrLockSta input boolean; ATAlarm output boolean; AntitheftSta output uint8; TailgateRemote output uint8; HornCtrl output boolean; VIG_Cmd input uint8 [0..7]; VehSpeed input single [0..1]; fVIGHandle input boolean; VBCM_FlashAntitheft_enum input uint8; fFirst local boolean; fHornOFF local boolean; AntitheftSeatFlod output boolean; APSOpenPTG input boolean; ENUM_ANTITHEFT_ALARM parameter uint8; ENUM_ANTITHEFT_ARM parameter uint8; VINP_FlashCountAlarm_enum input uint8; VINP_CANMsgValidGWZoneDR1_flg input boolean; VINP_CANMsgValidGWZoneFR1_flg input boolean; PcmdBuf local uint8; CountAlarm output uint8; IVI_Lock_SoundSW_Sta input boolean; VBCM_ATCtrl_enum output uint8; VBCM_LockAlarm_enum output uint8
  data PwrSta settings: description=Min=0, Max=2047, Engineering Unit = km/h, Offset=0 km/h, Resolution= 0.125 km/h per bit, >2047 = Invalid (bit 12 = 1)
  events: eLampLock local FUNCTION_CALL_EVENT; eLampUnlock local FUNCTION_CALL_EVENT; eLockAlert local FUNCTION_CALL_EVENT; eLock local FUNCTION_CALL_EVENT; eUnlock local FUNCTION_CALL_EVENT; eDoorOpen local FUNCTION_CALL_EVENT; eForceDisarm local FUNCTION_CALL_EVENT; eTailgate local FUNCTION_CALL_EVENT; eHornAlarm local FUNCTION_CALL_EVENT; eHornLock local FUNCTION_CALL_EVENT; eKeyIN local FUNCTION_CALL_EVENT; eLockFail local FUNCTION_CALL_EVENT; eActLock local FUNCTION_CALL_EVENT; eActUnlock local FUNCTION_CALL_EVENT; eTailgateRemote local FUNCTION_CALL_EVENT; eTailgateHandle local FUNCTION_CALL_EVENT; eTailgateReject local FUNCTION_CALL_EVENT

== stateflow chart bcm/BCM/BCM/CenterDoorLock/Chart ==
  settings: updateMethod=DISCRETE
  state ChargingDoor [parallel]
    settings: executionOrder=2
    state ChargingDoorUnlock
      en:FrChargingDoorCtrl=0;
      RrChargingDoorCtrl=0;
      FuelDoorPos=0;
    state U2L
      en:FrChargingDoorCtrl=2;
      RrChargingDoorCtrl=2;
    note: 100ms
    note: 100ms
    state L2U
      en:FrChargingDoorCtrl=1;
      RrChargingDoorCtrl=1;
    state ChargingDoorLock
      en:FrChargingDoorCtrl=0;
      RrChargingDoorCtrl=0;
      FuelDoorPos=1;
    (default) -> (junction 1986)
    (junction 1986) -> (junction 1988) [order 2]
    (junction 1986) -> ChargingDoorUnlock [order 1] : [!EEP_FuelDoorPos]
    (junction 1988) -> ChargingDoorLock
    ChargingDoorUnlock -> U2L : [AntitheftSta==1||AntitheftSta==3]
    L2U -> ChargingDoorUnlock : [after(10,tick)]
    U2L -> ChargingDoorLock : [after(10,tick)]
    ChargingDoorLock -> L2U : [AntitheftSta==0||AntitheftSta==2]
  state Unlock_Single_Setting [parallel]
    settings: executionOrder=1
    state Press
    state Release
      ex:LockSetting=!LockSetting;
    (default) -> Unlock_Single_Setting.Press : {LockSetting=EEP_LockSetting;}
    Unlock_Single_Setting.Press -> Unlock_Single_Setting.Release : [SetUnlockSingle==0]
    Unlock_Single_Setting.Release -> Unlock_Single_Setting.Press : [SetUnlockSingle==1]
  state CrashDetect [parallel]
    settings: executionOrder=9
    state OFF [commented out]
    state KeyON [commented out]
      state Initial [commented out]
        en:
        CrashDetd=0;
      state sCrash [commented out]
        en:CrashDetd=1;Unlockreq=1;
      note: 750 ms
      state Detect [commented out]
      Initial -> Detect [commented out] : [after(75,tick)]
      Detect -> sCrash [commented out] : [CrashOutputSts>0||....
          | (CrashInputFreq>4.1&&....
          | CrashInputFreq<4.2&&....
          | CrashInputDuty>16&&....
          | CrashInputDuty<17)]
    (default) -> CrashDetect.OFF [commented out]
    CrashDetect.OFF -> Initial [commented out] : [PwrSta>3]
    KeyON -> CrashDetect.OFF [commented out] : [PwrSta<=3]
    (default) -> (junction 1980)
    (junction 1980) -> (junction 1981) : [hasChanged(CrashDetd)]
    CrashDetect -> (junction 1980)
    (junction 1981) -> (junction 1979) : {Unlockreq=1;}
  state CentralDoorLockSW [parallel]
    settings: executionOrder=3
    state Release
    state Press
    (default) -> CentralDoorLockSW.Press
    CentralDoorLockSW.Press -> CentralDoorLockSW.Release : [!CentralDoorLockSW]
    CentralDoorLockSW.Release -> (junction 1817) : [CentralDoorLockSW]
    (junction 1817) -> CentralDoorLockSW.Press [order 1] : [BCM_DoorLock_Sta]/{Main.eDUnlock;}
    (junction 1817) -> (junction 1821) [order 2]
    (junction 1821) -> CentralDoorLockSW.Press [order 1] : [AllDoorSW]/{Main.eDUnlock;}
    (junction 1821) -> (junction 1824) [order 2]
    (junction 1824) -> CentralDoorLockSW.Press [order 1] : [CrashDetd==1]{Main.eDUnlock;}
    (junction 1824) -> (junction 1827) [order 2]
    (junction 1827) -> CentralDoorLockSW.Press : {Main.eCTDLock;}
  state IVICentralDoorLockSW [parallel]
    settings: executionOrder=4
    state Release
    state Press
    (default) -> IVICentralDoorLockSW.Press
    IVICentralDoorLockSW.Press -> IVICentralDoorLockSW.Release : [CDL_Unlock_Butt==0&&CDL_Lock_Butt==0]
    IVICentralDoorLockSW.Release -> (junction 1950) [order 1] : [CDL_Lock_Butt==1]
    (junction 1950) -> IVICentralDoorLockSW.Press [order 1] : [BCM_DoorLock_Sta]/{Main.eDUnlock;}
    (junction 1950) -> (junction 1951) [order 2]
    (junction 1951) -> IVICentralDoorLockSW.Press [order 1] : [AllDoorSW]/{Main.eDUnlock;}
    (junction 1951) -> (junction 1952) [order 2]
    (junction 1952) -> IVICentralDoorLockSW.Press [order 1] : [CrashDetd==1]{Main.eDUnlock;}
    (junction 1952) -> (junction 1953) [order 2]
    (junction 1953) -> IVICentralDoorLockSW.Press : {Main.eCTDLock;}
    IVICentralDoorLockSW.Release -> IVICentralDoorLockSW.Press [order 2] : [CDL_Unlock_Butt==1]{Main.eDUnlock;}
  state ATLockCtrl [parallel]
    settings: executionOrder=5
    state LockSend
      en:fUnlockSingle=1;
    state NoCommand
    state UnlockSend
      en:fUnlockSingle=0;
    (default) -> NoCommand : {fUnlockSingle=VINP_FlashfUnlockSingle_flg;}
    NoCommand -> (junction 1862) [order 2] : [ATLockCtrl==1]
    (junction 1862) -> LockSend [order 1] : [CrashDetd==1]
    (junction 1862) -> (junction 1865) [order 2] : {Main.eDLock;}
    (junction 1865) -> LockSend [order 1] : [LockSetting]
    (junction 1865) -> (junction 1867) [order 2]
    (junction 1867) -> LockSend
    LockSend -> NoCommand : [ATLockCtrl!=1]
    NoCommand -> (junction 1870) [order 1] : [ATLockCtrl==2]
    (junction 1870) -> UnlockSend [order 1] : [LockSetting==0||fUnlockSingle==0]/{Main.eDUnlock;}
    (junction 1870) -> (junction 1872) [order 2]
    (junction 1872) -> UnlockSend : /{Main.eSUnlock;}
    UnlockSend -> NoCommand : [ATLockCtrl!=2]
  state Main [parallel]
    settings: executionOrder=6
    note: 350 ms
    state WaitForReverse
      en:CTDCtrl=0;
    state StandBy
      en:CTDCtrl=0;
    state DoorLock
      en:CTDCtrl=3;
    note: 100 ms
    state DrDoorUnlock
      en:CTDCtrl=1;
      fVIGHandle=0;
    note: Unlockreq
    state DoorUnlock
      en:CTDCtrl=2;
      fVIGHandle=0;
      ex:Unlockreq=0;
    (default) -> Main.StandBy
    Main.StandBy -> DoorLock [order 1] : eDLock
    DoorLock -> WaitForReverse [order 1] : [after(35,tick)]/{LED.eResetLED;}
    DoorLock -> WaitForReverse [order 2] : [Unlockreq]/{LED.eResetLED;}
    Main.StandBy -> DoorLock [order 5] : eCTDLock{fVIGHandle=1;}
    WaitForReverse -> Main.StandBy : [after(10,tick)]
    Main.StandBy -> DrDoorUnlock [order 2] : eSUnlock
    DrDoorUnlock -> WaitForReverse [order 1] : [after(35,tick)]
    DrDoorUnlock -> DoorUnlock [order 2] : eDUnlock
    DrDoorUnlock -> DoorUnlock [order 3] : [Unlockreq]
    DoorUnlock -> WaitForReverse : [after(35,tick)]
    Main.StandBy -> DoorUnlock [order 3] : eDUnlock
    Main.StandBy -> DoorUnlock [order 4] : [Unlockreq]
  state AutoLock [parallel]
    settings: executionOrder=8
    state ON
      state StandBy
      state AutoLock
        en:Main.eDLock;
      AutoLock.ON.StandBy -> AutoLock.ON.AutoLock : [AirBagFailCmd==0 && CrashDetd==0 && VehSpeed>10]
      AutoLock.ON.AutoLock -> AutoLock.ON.StandBy : [VehSpeed<=0&&AllDoorSW==1]
    state OFF
    (default) -> AutoLock.OFF
    AutoLock.OFF -> AutoLock.ON.StandBy : [funAuto]
    AutoLock.ON -> AutoLock.OFF : [!funAuto]
  state LED [parallel]
    settings: executionOrder=7
    state OFF
      en:DoorLockIND=0;
    state ON
      en:DoorLockIND=1;
    note: 10 sec
    state HoldON
      en:DoorLockIND=1;
    (default) -> LED.OFF
    LED.ON -> LED.OFF [order 1] : [BCM_DoorLock_Sta==0]
    LED.OFF -> LED.ON [order 1] : [PwrSta>3&&BCM_DoorLock_Sta==1]
    HoldON -> LED.OFF [order 1] : [after(1000,tick)||BCM_DoorLock_Sta==0]
    LED.OFF -> HoldON [order 2] : eResetLED[BCM_DoorLock_Sta==1]
    HoldON -> LED.ON [order 2] : [PwrSta>3]
    LED.ON -> HoldON [order 2] : [PwrSta<=3]
    HoldON -> HoldON [order 3] : eResetLED
  data: SetUnlockSingle input boolean; LockSetting output boolean =0; AntitheftSta input uint8 [..3]; FrChargingDoorCtrl output uint8 [0..2]; RrChargingDoorCtrl output uint8 [0..2]; AllDoorSW input boolean; PwrSta input uint8 [0..5]; CentralDoorLockSW input boolean; BCM_DoorLock_Sta input boolean; CTDCtrl output uint8 [0..3]; DoorLockIND output boolean; ATLockCtrl input uint8 [0..2]; AirBagFailCmd input boolean; VehSpeed input; funAuto input boolean; fVIGHandle output boolean; CDL_Unlock_Butt input boolean; CDL_Lock_Butt input boolean; Unlockreq local boolean; CrashDetd input boolean; VINP_FlashfUnlockSingle_flg input; FuelDoorPos output; EEP_FuelDoorPos input; EEP_LockSetting input; fUnlockSingle output boolean
  events: eDLock local FUNCTION_CALL_EVENT; eDUnlock local FUNCTION_CALL_EVENT; eSUnlock local FUNCTION_CALL_EVENT; eCTDLock local FUNCTION_CALL_EVENT; eResetLED local FUNCTION_CALL_EVENT

== stateflow chart bcm/BCM/BCM/Dimmer/Chart ==
  settings: sampleTime=StepSize
  state CANDimmerCMD [parallel]
    settings: executionOrder=1
    state sWait
    (default) -> sWait
    (junction 1680) -> sWait : [MFRD_N_Bright_Req<=100&&IVI_Status]/{Dimmer=20+MFRD_N_Bright_Req*0.8}
    (junction 1677) -> (junction 1680) [order 1]
    (junction 1677) -> sWait [order 2]
    (junction 1609) -> (junction 1677)
    sWait -> (junction 1609) : [after(20,tick)]
  state sDimmer_EN [parallel]
    settings: executionOrder=2  description=This state models the modes of a door sensor and implements logic to respond when that sensor is producing a signal.
    state sOFF
      en:DimmerEN=0;
    state sON
      en:DimmerEN=1;
    (default) -> sOFF
      settings: description=On the first sample call the door mode is set to active.
    sON -> sOFF : [!PLamp||IVI_Night_Mode_Sta]
    sOFF -> sON : [PLamp&&!IVI_Night_Mode_Sta]
  data: IVI_Status input boolean; IVI_Night_Mode_Sta input boolean; Dimmer output single =0; DimmerEN output boolean; PLamp input boolean; MFRD_N_Bright_Req input =0
  data IVI_Night_Mode_Sta settings: description=Min=0, Max=2047, Engineering Unit = km/h, Offset=0 km/h, Resolution= 0.125 km/h per bit, >2047 = Invalid (bit 12 = 1)
  data Dimmer settings: description=|
      | Bcm Buzzer output results.
      | 0 = None Buzzer
      | 1 = Turn signal Buzzer
      | 2 = Key Reminder Buzzer
      | 3 = Seat Belt Buzzer
      | 4 = Light Monitor Buzzer
